simulink model "Nomoto_simulink"  (R2020a)
settings: Solver=VariableStepAuto  StartTime=0.0  StopTime=1500  RelTol=1e-3
values from neighbouring files (symbols this model uses):
  A = [1, 0 ... (first row only)    [Nomoto.m]
  B = [y ... (first row only)    [Nomoto.m]
  C = eye(2)    [Nomoto.m]
libraries: simulink x3
settings Model: Creator=micro microndas  LastModifiedBy=micro microndas

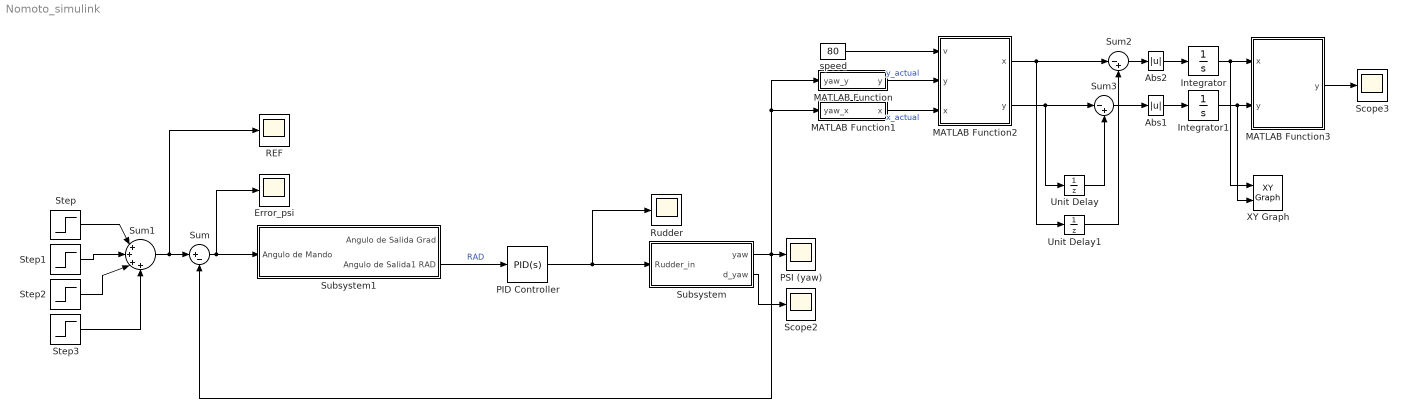
== system Nomoto_simulink ==
  Abs1 : Abs
  Abs2 : Abs
  Error_psi : Scope
  Integrator : Integrator
  Integrator1 : Integrator
  MATLAB Function : MATLAB Function  TreatAsAtomicUnit=on
  MATLAB Function1 : MATLAB Function  TreatAsAtomicUnit=on
  MATLAB Function2 : MATLAB Function  TreatAsAtomicUnit=on
  MATLAB Function3 : MATLAB Function  TreatAsAtomicUnit=on
  PID Controller : simulink/Continuous/PID Controller  Controller=PID  Form=Parallel  TimeDomain=Continuous-time  UseExternalTs=off  SampleTime=-1  IntegratorMethod=Forward Euler  FilterMethod=Forward Euler  ControllerParametersSource=internal  P=0.0577585797469675  I=1.00017165034907e-05  D=13.1187350392577  UseFilter=on  N=2.35835127099285  TunerSelectOption=Transfer Function Based (PID Tuner App)  InitialConditionSource=internal  InitialConditionForIntegrator=0  InitialConditionForFilter=0  DifferentiatorICPrevScaledInput=0  ExternalReset=none  TrackingMode=off  Kt=1  LimitOutput=off  UpperSaturationLimit=inf  LowerSaturationLimit=-inf  LinearizeAsGain=on  AntiWindupMode=none  Kb=1  POutMin=[]  POutMax=[]  IOutMin=[]  IOutMax=[]  DOutMin=[]  DOutMax=[]  NOutMin=[]  NOutMax=[]  SumOutMin=[]  SumOutMax=[]  SaturationOutMin=[]  SaturationOutMax=[]  PParamMin=[]  PParamMax=[]  IParamMin=[]  IParamMax=[]  DParamMin=[]  DParamMax=[]  NParamMin=[]  NParamMax=[]  KbParamMin=[]  KbParamMax=[]  KtParamMin=[]  KtParamMax=[]  KbOutMin=[]  KbOutMax=[]  KtOutMin=[]  KtOutMax=[]  IntegratorOutMin=[]  IntegratorOutMax=[]  FilterOutMin=[]  FilterOutMax=[]  SumI1OutMin=[]  SumI1OutMax=[]  SumI2OutMin=[]  SumI2OutMax=[]  SumI3OutMin=[]  SumI3OutMax=[]  SumI4OutMin=[]  SumI4OutMax=[]  SumDOutMin=[]  SumDOutMax=[]  DifferentiatorOutMin=[]  DifferentiatorOutMax=[]  FilterDiffOutCoefMin=[]  FilterDiffOutCoefMax=[]  ReciprocalOutMin=[]  ReciprocalOutMax=[]  SumDenOutMin=[]  SumDenOutMax=[]  SumNumOutMin=[]  SumNumOutMax=[]  DivideOutMin=[]  DivideOutMax=[]  UdiffTsProdOutMin=[]  UdiffTsProdOutMax=[]  NTsProdOutMin=[]  NTsProdOutMax=[]  UintegralTsProdOutMin=[]  UintegralTsProdOutMax=[]  UngainTsProdOutMin=[]  UngainTsProdOutMax=[]  IntegratorContinuousStateAttributes=''  IntegratorStateMustResolveToSignalObject=off  IntegratorRTWStateStorageClass=Auto  FilterContinuousStateAttributes=''  FilterStateMustResolveToSignalObject=off  FilterRTWStateStorageClass=Auto  ParallelPVariant=InternalParameters  IdealPVariant=Disabled  IVariant=InternalParameters  DVariant=InternalParameters  IntegratorVariant=Continuous  SatVariant=Disabled  AWVariant=Passthrough  PCopyVariant=Disabled  TRVariant=Disabled  FdbkBlocksVariant=Forward  IdealPFdbkVariant=Disabled  SatFdbkVariant=Disabled  DerivativeFilterVariant=ContFilter  NVariant=InternalParameters  NCopyVariant=Disabled  FilterICVariant=InternalICsFilter  IntegratorICVariant=InternalICs  ExternalResetVariant=Disabled  TRSumVariant=Passthrough  SumFdbkVariant=Disabled  SumVariant=Sum_PID  TsampFilterVariant=InternalTs  TsampNgainVariant=Passthrough  TsampIntegralVariant=Passthrough
  PSI (yaw) : Scope
  REF : Scope
  Rudder : Scope
  Scope2 : Scope
  Scope3 : Scope
  Step : Step  Time=100  Before=0.2  After=0  SampleTime=0
  Step1 : Step  Time=500  After=0.12  SampleTime=0
  Step2 : Step  Time=800  After=0  SampleTime=0
  Step3 : Step  Time=1200  After=-0.15  SampleTime=0
  Subsystem : Subsystem
  Subsystem1 : Subsystem
  Sum : Sum  Inputs=|+-
  Sum1 : Sum  Inputs=|++++
  Sum2 : Sum  Inputs=|-+
  Sum3 : Sum  Inputs=|-+
  Unit Delay : UnitDelay  SampleTime=-1  HasFrameUpgradeWarning=on
  Unit Delay1 : UnitDelay  SampleTime=-1  HasFrameUpgradeWarning=on
  XY Graph : simulink/Sinks/XY Graph  xmin=-20  xmax=20  ymin=-20  ymax=20  st=0.1
  speed : Constant  Value=80
  wires:
  Sum1/1 -> REF/1, Sum/1
  Subsystem1/2(Angulo de Salida1 RAD) -> PID Controller/1  "RAD"
  Subsystem/1(yaw) -> MATLAB Function1/1(yaw_x), MATLAB Function/1(yaw_y), PSI (yaw)/1, Sum/2
  Sum/1 -> Error_psi/1, Subsystem1/1(Angulo de Mando)
  Subsystem/2(d_yaw) -> Scope2/1
  Step/1 -> Sum1/1
  PID Controller/1 -> Rudder/1, Subsystem/1(Rudder_in)
  Step2/1 -> Sum1/3
  Step1/1 -> Sum1/2
  Unit Delay1/1 -> Sum2/2
  Integrator1/1 -> XY Graph/2, MATLAB Function3/2("y ")
  MATLAB Function3/1(y) -> Scope3/1
  MATLAB Function2/2(y) -> Unit Delay/1, Sum3/1
  Integrator/1 -> XY Graph/1, MATLAB Function3/1(x)
  Unit Delay/1 -> Sum3/2
  MATLAB Function2/1(x) -> Unit Delay1/1, Sum2/1
  MATLAB Function/1(y) -> MATLAB Function2/2("y ")  "y_actual"
  MATLAB Function1/1(x) -> MATLAB Function2/3("x ")  "x_actual"
  speed/1 -> MATLAB Function2/1(v)
  Sum3/1 -> Abs1/1
  Abs1/1 -> Integrator1/1
  Sum2/1 -> Abs2/1
  Abs2/1 -> Integrator/1
  Step3/1 -> Sum1/4

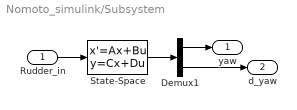
== system Nomoto_simulink/Subsystem ==
  Rudder_in : Inport
  Demux1 : Demux  Outputs=2
  State-Space : StateSpace  A=A  B=B  C=C  D=[0;0]  InitialCondition=0  ContinuousStateAttributes={'yaw','d_yaw'}
  yaw : Outport
  d_yaw : Outport  Port=2
  wires:
  Rudder_in/1 -> State-Space/1
  State-Space/1 -> Demux1/1
  Demux1/1 -> yaw/1
  Demux1/2 -> d_yaw/1

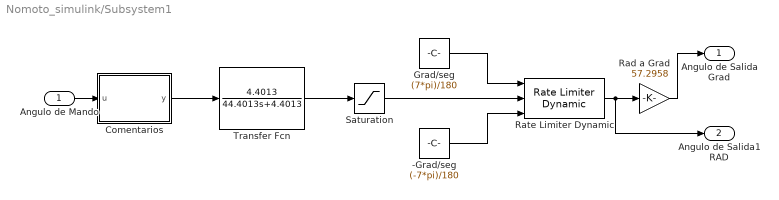
== system Nomoto_simulink/Subsystem1 ==
  Angulo de Mando : Inport
  -Grad/seg : Constant  Value=(-7*pi)/180
  Comentarios : MATLAB Function  TreatAsAtomicUnit=on
  Grad/seg : Constant  Value=(7*pi)/180
  Rad a Grad : Gain  Gain=57.2958
  Rate Limiter Dynamic : simulink/Discontinuities/Rate Limiter Dynamic
  Saturation : Saturate  UpperLimit=pi/6  LowerLimit=-pi/6
  Transfer Fcn : TransferFcn  Numerator=[4.4013]  Denominator=[44.4013 4.4013]
  Angulo de Salida Grad : Outport
  Angulo de Salida1 RAD : Outport  Port=2
  wires:
  Grad/seg/1 -> Rate Limiter Dynamic/1
  -Grad/seg/1 -> Rate Limiter Dynamic/3
  Rate Limiter Dynamic/1 -> Angulo de Salida1 RAD/1, Rad a Grad/1
  Rad a Grad/1 -> Angulo de Salida Grad/1
  Comentarios/1(y) -> Transfer Fcn/1
  Angulo de Mando/1 -> Comentarios/1(u)
  Transfer Fcn/1 -> Saturation/1
  Saturation/1 -> Rate Limiter Dynamic/2

== matlab function Nomoto_simulink/MATLAB Function ==
  data: yaw_y input; y output
function y = fcn(yaw_y)

y = sin(yaw_y);

== matlab function Nomoto_simulink/Subsystem1/Comentarios ==
  data: u input; y output
function y = fcn(u)

%Kg' = Kg*L / U
    %Kg = Maximo giro del timon / error maximo
        %error maximo
        %Maximo giro del timon
    %L = Eslora / Longitud del buque
        %390.00 𝑓𝑡 
        %118.872 mts
    %U = Velocidad del buque
        %15 nudo nautico
        %7.7166 m/s

y = u;

== matlab function Nomoto_simulink/MATLAB Function1 ==
  data: yaw_x input; x output
function x = fcn(yaw_x)

x = cos(yaw_x);

== matlab function Nomoto_simulink/MATLAB Function2 ==
  data: x output; v input; y output; y input; x input
function [x,y] = fcn(v,y,x)
x = v*x;
y = v*y;

== matlab function Nomoto_simulink/MATLAB Function3 ==
  data: x input; y output; y input
function y = fcn(x,y)

y = atan(y/x);
